simulink model "kapitza_manual_model2"  (R2025b)
settings: Solver=ode45  StartTime=0.0  StopTime=20  MaxStep=0.00012566370614359171  RelTol=1e-7  AbsTol=1e-9
values from neighbouring files (symbols this model uses):
  p = [g; L; zeta; A; f]    [kapitza_controle.m]    (also in parameters_kapitza_model2.m)
  x0 = [150*pi/180; 0]    [kapitza_controle.m]    (also in parameters_kapitza_model2.m = [45*pi/180; 0])
libraries: simulink x1
settings Model: Creator=rafae  LastModifiedBy=rafae
settings SolverCC: AutoScaleAbsTol=off

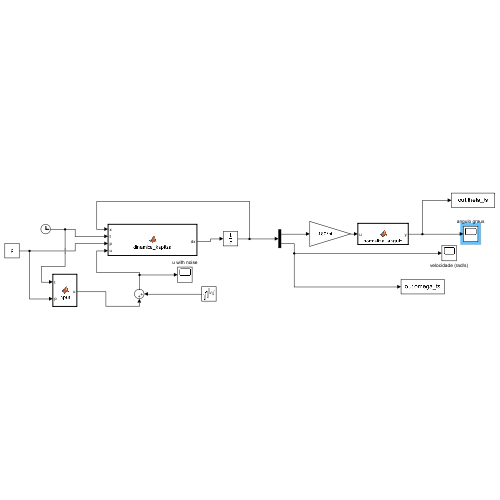
[thumbnail: Simulink's stored preview of the top-level diagram]
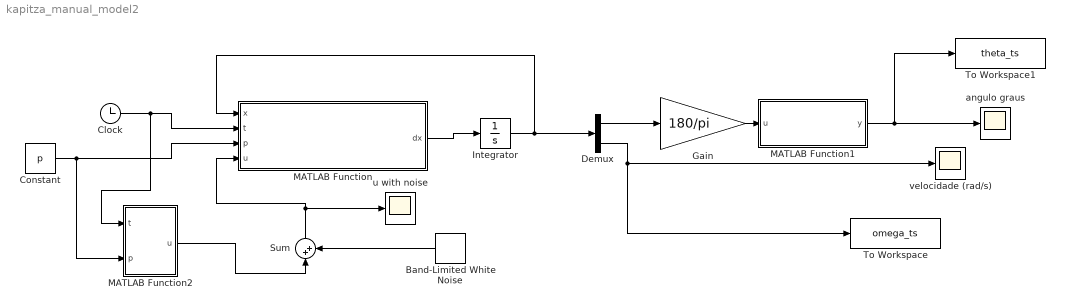
== system kapitza_manual_model2 ==
  Band-Limited White Noise : simulink/Sources/Band-Limited White Noise  Cov=[5]  Ts=0.1  seed=[23341]
  Clock : Clock
  Constant : Constant  Value=p
  Demux : Demux  Outputs=2
  Gain : Gain  Gain=180/pi
  Integrator : Integrator  InitialCondition=x0
  MATLAB Function : MATLAB Function  TreatAsAtomicUnit=on
  MATLAB Function1 : MATLAB Function  TreatAsAtomicUnit=on
  MATLAB Function2 : MATLAB Function  TreatAsAtomicUnit=on
  Sum : Sum  Inputs=|++
  To Workspace : ToWorkspace  VariableName=omega_ts  SaveFormat=Timeseries  SampleTime=-1
  To Workspace1 : ToWorkspace  VariableName=theta_ts  SaveFormat=Timeseries  SampleTime=-1
  angulo graus : Scope
      settings: ActiveDisplayYMinimum=-224.99999940303155  ActiveDisplayYMaximum=224.99999902335452
  u with noise : Scope
      settings: ActiveDisplayYMinimum=-2257.7856330249774  ActiveDisplayYMaximum=2262.7151381629615  DataLoggingVariableName=ScopeData2
  velocidade (rad/s) : Scope
      settings: ActiveDisplayYMinimum=-1  ActiveDisplayYMaximum=1
  wires:
  Clock/1 -> MATLAB Function2/1(t), MATLAB Function/2(t)
  Constant/1 -> MATLAB Function2/2(p), MATLAB Function/3(p)
  MATLAB Function/1(dx) -> Integrator/1
  Integrator/1 -> MATLAB Function/1(x), Demux/1
  Demux/2 -> velocidade (rad/s)/1, To Workspace/1
  Gain/1 -> MATLAB Function1/1(u)
  Demux/1 -> Gain/1
  MATLAB Function1/1(y) -> To Workspace1/1, angulo graus/1
  Sum/1 -> u with noise/1, MATLAB Function/4(u)
  Band-Limited White Noise/1 -> Sum/2
  MATLAB Function2/1(u) -> Sum/1

== matlab function kapitza_manual_model2/MATLAB Function1 ==
  data: u input; y output
function y = normaliza_angulo(u)
    y = mod(u + 180, 360) - 180;
end

== matlab function kapitza_manual_model2/MATLAB Function ==
  data: x input; dx output; t input; p input; u input
function dx = dinamica_kapitza(x, t, p, u)
%#codegen

g = p(1);
L = p(2);
zeta = p(3);
A = p(4);
f = p(5);

theta = x(1);
velocidade = x(2);

wn = sqrt(g/L);
% w = 2*pi*f;
% 
% u = A*w^2*cos(w*t);

dx = zeros(2,1);
dx(1) = velocidade;

dx(2) = -2*zeta*wn*velocidade ...
        + (g/L-u/L)*sin(theta);
end

== matlab function kapitza_manual_model2/MATLAB Function2 ==
  data: u output; t input; p input
function u = input(t, p)
%#codegen

A = p(4);
f = p(5);

w = 2*pi*f;

u = A*w^2*cos(w*t);

end
